simulink model "simBandLtdWN"  (R2020a)
settings: Solver=FixedStepAuto  StartTime=0.0  StopTime=1  FixedStep=1e-5  RelTol=1e-3
libraries: simulink_extras x1, simulink x1, commseqgen3 x1
settings Model: Creator=胡子瀚  LastModifiedBy=胡子瀚

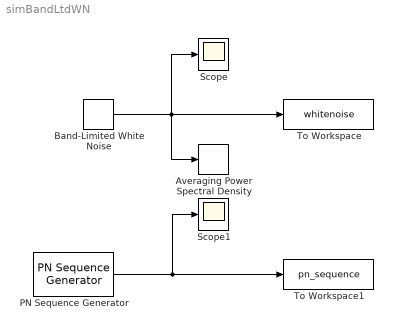
== system simBandLtdWN ==
  Averaging Power Spectral Density : simulink_extras/Additional Sinks/Averaging Power Spectral Density  npts=128  fftpts=512  HowOften=64  sampleT=0.001
      settings: SourceProductBaseCode=SL
  Band-Limited White Noise : simulink/Sources/Band-Limited White Noise  Cov=0.001  Ts=1e-4  seed=23341
  PN Sequence Generator : commseqgen3/PN Sequence Generator  poly=[1 0 1 0 0 1]  ini_sta=[0 0 0 0 1]  outBitMaskSource=Dialog parameter  shift=0  outVarSiz=off  maxOutSizeMode=Dialog parameter  maxOutSize=[10 1]  Ts=0.0001  sampPerFrame=1  reset=off  bitPackedOutputs=off  outDataType=double  numPackedBits=8  bitPackDataSigned=off  bitPackedOutDType=double
  Scope : Scope
  Scope1 : Scope
  To Workspace : ToWorkspace  VariableName=whitenoise  SampleTime=-1
  To Workspace1 : ToWorkspace  VariableName=pn_sequence  SampleTime=-1
  wires:
  Band-Limited White Noise/1 -> Averaging Power Spectral Density/1, Scope/1, To Workspace/1
  PN Sequence Generator/1 -> Scope1/1, To Workspace1/1
